simulink model "lab3_sim"  (R2023b)
settings: Solver=FixedStepAuto  StartTime=0.0  StopTime=10.0  FixedStep=0.001  RelTol=1e-4  EnableMultiTasking=on
values from neighbouring files (symbols this model uses):
  a = [1 -0.593500566074 0.909216960138 -0.294350243957 0.149045009629 -0.0204654325002 0.00247640676414]    [aggresive_slanted.mat]    (also in aggressive.mat; normal.mat; normal_slanted.mat)
  b = [0.0180065958438 0.108039575063 0.270098937656 0.360131916875 0.270098937656 0.108039575063 0.0180065958438]    [aggresive_slanted.mat]    (also in aggressive.mat; normal.mat; normal_slanted.mat)
undefined symbols (not defined in the file or in its folder): K, theta, TI, VMAX_UPM
settings Model: Creator=maggiore  LastModifiedBy=xiaom
settings SolverCC: AlgebraicLoopSolver=TrustRegion
settings DataIOCC: LimitDataPoints=on  SaveFormat=Array  SignalLoggingSaveFormat=ModelDataLogs  ReturnWorkspaceOutputs=off
settings OptimizationCC: ExpressionDepthLimit=2147483647  InitFltsAndDblsToZero=on  LifeSpan=inf
settings DebuggingCC: SaveWithParameterizedLinksMsg=none  UnderspecifiedInitializationDetection=Classic  MergeDetectMultiDrivingBlocksExec=none  SignalResolutionControl=TryResolveAllWithWarning  SolverPrmCheckMsg=warning  MultiTaskDSMMsg=warning  MultiTaskCondExecSysMsg=none  FcnCallInpInsideContextMsg=warning  UnconnectedInputMsg=warning  UnconnectedOutputMsg=warning  UnconnectedLineMsg=warning  StateNameClashWarn=warning  SFUnexpectedBacktrackingDiag=warning  SFNoUnconditionalDefaultTransitionDiag=warning  SFExecutionAtInitializationDiag=none  ArithmeticOperatorsInVariantConditions=warning
settings HardwareCC: ProdBitPerPointer=32  ProdBitPerSizeT=32  ProdBitPerPtrDiffT=32  ProdLargestAtomicFloat=None  ProdIntDivRoundTo=Undefined  ProdEndianess=Unspecified  ProdWordSize=32  ProdHWDeviceType=32-bit Generic
settings ModelReferenceCC: PropagateSignalLabelsOutOfModel=off
settings SFSimCC: SimUseLocalCustomCode=off  CustomCodeUndefinedFunction=UseInterfaceOnly
settings RTWCC: RTWUseLocalCustomCode=off
settings CodeAppCC: StateflowObjectComments=on
settings GRTTargetCC: TargetFcnLib=ansi_tfl_tmw.mat  TargetLangStandard=C89/C90 (ANSI)  CombineOutputUpdateFcns=off  GRTInterface=on
settings ConfigComp: CovMetricSettings=dw  CovSaveCumulativeToWorkspaceVar=on  CovSaveSingleToWorkspaceVar=on  CovExternalEMLEnable=off

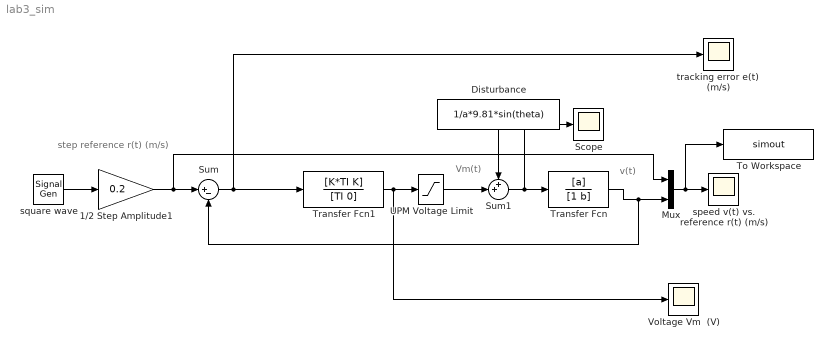
== system lab3_sim ==
  note: step reference r(t) (m/s)
  note: Vm(t)
  note: v(t)
  1/2 Step Amplitude1 : Gain  Gain=0.2  SaturateOnIntegerOverflow=on  OutDataTypeStr=Inherit: Same as input  ParamDataTypeStr=Inherit: Same as input
  Disturbance : Constant  Value=1/a*9.81*sin(theta)
  Mux : Mux  Inputs=2
  Scope : Scope
  Sum : Sum  Inputs=|+-
  Sum1 : Sum  Inputs=++|
  To Workspace : ToWorkspace  VariableName=simout  SaveFormat=Timeseries  SampleTime=-1
  Transfer Fcn : TransferFcn  Numerator=[a]  Denominator=[1 b]
  Transfer Fcn1 : TransferFcn  Numerator=[K*TI K]  Denominator=[TI 0]
  UPM Voltage Limit : Saturate  UpperLimit=VMAX_UPM  LowerLimit=- VMAX_UPM
  Voltage Vm  (V) : Scope
  speed v(t) vs. reference r(t) (m/s) : Scope
  square wave : SignalGenerator  WaveForm=square  Frequency=.5
  tracking error e(t)  (m/s) : Scope
  wires:
  Sum/1 -> tracking error e(t)  (m/s)/1, Transfer Fcn1/1
  square wave/1 -> 1/2 Step Amplitude1/1
  Mux/1 -> To Workspace/1, speed v(t) vs. reference r(t) (m/s)/1
  Transfer Fcn1/1 -> UPM Voltage Limit/1, Voltage Vm  (V)/1
  Sum1/1 -> Scope/1, Transfer Fcn/1
  Disturbance/1 -> Sum1/1
  1/2 Step Amplitude1/1 -> Sum/1, Mux/1
  UPM Voltage Limit/1 -> Sum1/2
  Transfer Fcn/1 -> Mux/2, Sum/2
